simulink model "experimental_results"  (Simulink 10.2)
settings: Solver=ode1  StartTime=0.0  StopTime=60  FixedStep=0.002  RelTol=1e-3  EnableMultiTasking=on
PreLoadFcn:
  | quanser_aero_lqr
undefined symbols (not defined in the file or in its folder): HIL, qc_get_step_size
libraries: quarc_library x7
(part 1 of 2)
settings Model: Creator=MLevis  LastModifiedBy=ffsandva  SimulationMode=external  ExtModeTrigDuration=20000
settings SolverCC: PositivePriorityOrder=on
settings DataIOCC: LimitDataPoints=on  SignalLoggingSaveFormat=Dataset
settings DebuggingCC: UnderspecifiedInitializationDetection=Simplified  MergeDetectMultiDrivingBlocksExec=error  SolverPrmCheckMsg=warning  FcnCallInpInsideContextMsg=error
settings RTWCC: Description=QUARC Win64 Target  SystemTargetFile=quarc_win64.tlc  TemplateMakefile=quarc_default_tmf
settings STFCustomTargetCC: TargetPreCompLibLocation=C:\PROGRA~3\QUARC\lib\2020b\win64\release  ConcurrentExecutionCompliant=on  SystemTargetFile=quarc_win64.tlc
settings GRTTargetCC: TargetPreCompLibLocation=C:\PROGRA~3\QUARC\lib\2020b\win64\release  ParMdlRefBuildCompliant=off  CompOptLevelCompliant=off  MatFileLogging=off  CPPClassGenCompliant=off  UseToolchainInfoCompliant=off  ExtMode=on  ExtModeMexFile=quarc_comm
settings ConfigComp: CovSFcnEnable=off

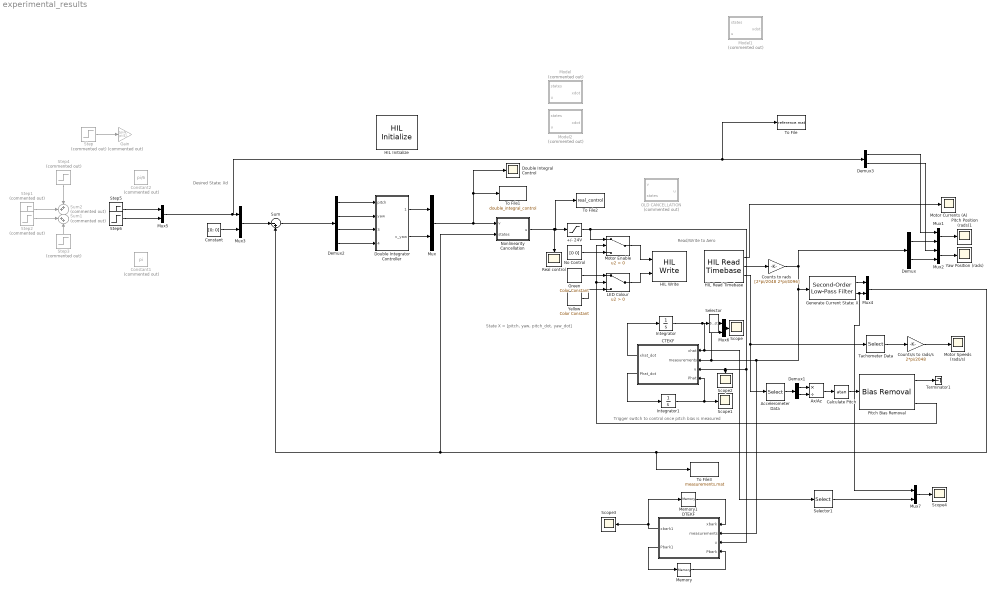
== system experimental_results ==
  note: Read/Write to Aero
  note: Trigger switch to control once pitch bias is measured
  note: Desired State; Xd
  note: State X = [pitch, yaw, pitch_dot, yaw_dot]
  +/- 24V : Saturate  UpperLimit=24  LowerLimit=-24
  Accelerometer Data : Selector  InputPortWidth=4  IndexOptions=Index vector (dialog)  Indices=[1 2]  OutputSizes=1
  Ax/Az : Product  Inputs=*/
  CTEKF : MATLAB Function  TreatAsAtomicUnit=on
  Calculate Pitch : Trigonometry  Operator=atan
  Constant : Constant  Value=[0; 0]
  Constant1 : Constant  Commented=on  Value=pi
  Constant2 : Constant  Commented=on  Value=pi/6
  Counts to rads : Gain  Gain=[2*pi/2048 2*pi/4096]
  Counts/s to rads/s : Gain  Gain=2*pi/2048
  DTEKF : MATLAB Function  TreatAsAtomicUnit=on
  Demux : Demux  Outputs=2
  Demux1 : Demux  Outputs=2
  Demux2 : Demux
  Demux3 : Demux  Outputs=2
  Double Integral Control : Scope
  Double Integrator Controller : Subsystem
  Gain : Gain  Commented=on  Gain=[pi/6; pi/4]
  Generate Current State; X : quarc_library/Continuous/Second-Order Low-Pass Filter  params_source=Internal (dialog parameters)  input_width=50  input_zeta=0.8  input_init=0
  Green : quarc_library/Sources/Signals/Color Constant  color=[0 1 0]
      settings: SourceProductName=QUARC Targets
  HIL Initialize : quarc_library/Data Acquisition/Generic/Configuration/HIL Initialize  Priority=-99  object_name=HIL-1  board_type=quanser_aero_usb  board_number=0  board_options=""  exclusive=off  active=off  hardware_clocks=[0]  clock_modes=[]  initial_clock_frequencies=[]  set_clock_params_at_start=off  set_clock_params_at_switch_in=off  set_clock_frequencies_at_start=off  set_clock_frequencies_at_switch_in=off  analog_input_channels=[0:1]  analog_input_configurations=[]  analog_input_maximums=3  analog_input_minimums=-3  set_analog_input_params_at_start=off  set_analog_input_params_at_switch_in=off  analog_output_channels=[0:1]  analog_output_maximums=24  analog_output_minimums=-24  initial_analog_outputs=[0]  final_analog_outputs=[0]  watchdog_analog_outputs=[0]  set_analog_output_params_at_start=off  set_analog_output_params_at_switch_in=off  set_analog_outputs_at_start=on  set_analog_outputs_at_switch_in=off  set_analog_outputs_at_terminate=on  set_analog_outputs_at_switch_out=off  set_analog_outputs_on_watchdog=on  digital_input_channels=[]  digital_output_channels=[0:1]  digital_output_configuration=[]  initial_digital_outputs=[1]  final_digital_outputs=[0]  watchdog_digital_outputs=[0]  set_digital_output_params_at_start=off  set_digital_output_params_at_switch_in=off  set_digital_outputs_at_start=on  set_digital_outputs_at_switch_in=off  set_digital_outputs_at_terminate=on  set_digital_outputs_at_switch_out=off  set_digital_outputs_on_watchdog=on  encoder_channels=[0:3]  quadrature=[4]  encoder_filter_frequency=[]  initial_encoder_counts=[0]  set_encoder_params_at_start=off  set_encoder_params_at_switch_in=off  set_encoder_counts_at_start=on  set_encoder_counts_at_switch_in=off  pwm_channels=[]  pwm_modes=[]  pwm_frequency=[]  pwm_configuration=[]  pwm_alignment=[]  pwm_polarity=[]  pwm_leading_deadband=[]  pwm_trailing_deadband=[]  initial_pwm_outputs=[]  final_pwm_outputs=[]  watchdog_pwm_outputs=[]  set_pwm_params_at_start=off  set_pwm_params_at_switch_in=off  set_pwm_outputs_at_start=off  set_pwm_outputs_at_switch_in=off  set_pwm_outputs_at_terminate=off  set_pwm_outputs_at_switch_out=off  set_pwm_outputs_on_watchdog=off  other_output_channels=[11000:11002]  initial_other_outputs=[0 1 0]  final_other_outputs=[1 0 0]  watchdog_other_outputs=[0 0 1]  set_other_outputs_at_start=on  set_other_outputs_at_switch_in=off  set_other_outputs_at_terminate=on  set_other_outputs_at_switch_out=off  set_other_outputs_on_watchdog=on
  HIL Read Timebase : quarc_library/Data Acquisition/Generic/Timebases/HIL Read Timebase  object_name=HIL-1  clock=0  analog_channels=[0:1]  encoder_channels=[2:3]  digital_channels=[]  other_channels=[4000 4002 14000 14001]  active=on  vector_output=on  data_type_mode=Inherit via back propagation  encoder_data_type=double  digital_data_type=boolean  overflow_mode=Error on overflow  samples_in_buffer=max(ceil(1/qc_get_step_size), 1)
  HIL Write : quarc_library/Data Acquisition/Generic/Immediate I//O/HIL Write  object_name=HIL-1  analog_channels=[0:1]  pwm_channels=[]  digital_channels=[]  other_channels=[11000:11002]  sample_time=-1  active=off  vector_input=on
  Integrator : Integrator  InitialCondition=[0;0;0;0]
  Integrator1 : Integrator  InitialCondition=zeros(4)
  LED Colour : Switch  Criteria=u2 > Threshold
  Memory : Memory  InitialCondition=zeros(4)
  Memory1 : Memory  InitialCondition=zeros(4,1)
  Model : MATLAB Function  Commented=on  TreatAsAtomicUnit=on
  Model1 : MATLAB Function  Commented=on  TreatAsAtomicUnit=on
  Model2 : MATLAB Function  Commented=on  TreatAsAtomicUnit=on
  Motor Currents (A) : Scope
  Motor Enable : Switch  Criteria=u2 > Threshold
  Motor Speeds (rads/s) : Scope
  Mux{,1..7} (8 alike) : Mux  Inputs=2
  No Control : Constant  Value=[0 0]
  Nonlinearity Cancellation : MATLAB Function  TreatAsAtomicUnit=on
  OLD CANCELLATION : MATLAB Function  Commented=on  TreatAsAtomicUnit=on
  Pitch Bias Removal : quarc_library/Discrete/Bias Removal  start_time=0  end_time=1  switch_id=0  sample_time=qc_get_step_size
      settings: SourceProductName=QUARC Targets
  Pitch Position (rads)1 : Scope
  Real control : Scope
  Scope{,1..4} (5 alike) : Scope
  Selector : Selector  InputPortWidth=4  IndexOptions=Index vector (dialog)  Indices=[1 2]  OutputSizes=1
  Selector1 : Selector  InputPortWidth=4  IndexOptions=Index vector (dialog)  Indices=[3 4]  OutputSizes=1
  Step : Step  Commented=on  Time=5  SampleTime=0
  Step1 : Step  Commented=on  Time=5  After=pi/6  SampleTime=0
  Step2 : Step  Commented=on  Time=5  After=-pi/2  SampleTime=0
  Step3 : Step  Commented=on  Time=30  After=pi/2  SampleTime=0
  Step4 : Step  Commented=on  Time=20  After=-pi/3  SampleTime=0
  Step5 : Step  Time=5  After=pi/6  SampleTime=0
  Step6 : Step  Time=5  After=pi/4  SampleTime=0
  Sum : Sum  Inputs=|-+
  Sum1 : Sum  Commented=on  Inputs=|++
  Sum2 : Sum  Commented=on  Inputs=++|
  Tachometer Data : Selector  InputPortWidth=4  IndexOptions=Index vector (dialog)  Indices=[3 4]  OutputSizes=1
  Terminator1 : Terminator
  To File : ToFile  Filename=reference.mat
  To File1 : ToFile  Filename=double_integral_control
  To File2 : ToFile  Filename=real_control
  To File3 : ToFile  Filename=measurements.mat
  Yaw Position (rads) : Scope
  Yellow : quarc_library/Sources/Signals/Color Constant  color=[1 1 0]
      settings: SourceProductName=QUARC Targets
  wires:
  HIL Read Timebase/2 -> Counts to rads/1
  +/- 24V/1 -> DTEKF/3(u), CTEKF/3(u), Scope2/1, Motor Enable/1
  Motor Enable/1 -> HIL Write/1
  Pitch Bias Removal/3 -> Motor Enable/2, LED Colour/2
  LED Colour/1 -> HIL Write/2
  No Control/1 -> Motor Enable/3
  Green/1 -> LED Colour/1
  Yellow/1 -> LED Colour/3
  Counts to rads/1 -> Demux/1, DTEKF/2(measurements), Mux6/2, CTEKF/2(measurements), Generate Current State; X/1
  HIL Read Timebase/3 -> Accelerometer Data/1, Tachometer Data/1
  Demux1/1 -> Ax/Az/1
  Demux1/2 -> Ax/Az/2
  Ax/Az/1 -> Calculate Pitch/1
  Calculate Pitch/1 -> Pitch Bias Removal/1
  Pitch Bias Removal/1 -> Terminator1/1
  HIL Read Timebase/1 -> Motor Currents (A)/1
  Counts/s to rads/s/1 -> Motor Speeds (rads/s)/1
  Tachometer Data/1 -> Counts/s to rads/s/1
  Accelerometer Data/1 -> Demux1/1
  Generate Current State; X/2 -> Mux7/1, Mux4/2
  Generate Current State; X/1 -> Mux4/1
  Demux/1 -> Mux1/2
  Mux1/1 -> Pitch Position (rads)1/1
  Demux/2 -> Mux2/2
  Mux2/1 -> Yaw Position (rads)/1
  Mux4/1 -> Sum/2, Nonlinearity Cancellation/2(states), To File3/1
  Double Integrator Controller/1(v_pitch) -> Mux/1
  Double Integrator Controller/2(v_yaw) -> Mux/2
  Demux2/1 -> Double Integrator Controller/1(pitch)
  Demux2/2 -> Double Integrator Controller/2(yaw)
  Demux2/3 -> Double Integrator Controller/3(pitch_dot)
  Demux2/4 -> Double Integrator Controller/4(yaw_dot)
  Sum/1 -> Demux2/1
  Mux5/1 -> To File/1, Demux3/1, Mux3/1
  Constant/1 -> Mux3/2
  Mux3/1 -> Sum/1
  Demux3/1 -> Mux1/1
  Demux3/2 -> Mux2/1
  Mux/1 -> Nonlinearity Cancellation/1(v), Double Integral Control/1, To File1/1
  Step/1 -> Gain/1
  Step2/1 -> Sum1/1
  Step1/1 -> Sum2/2
  Step3/1 -> Sum1/2
  Step4/1 -> Sum2/1
  Nonlinearity Cancellation/1(u) -> Real control/1, To File2/1, +/- 24V/1
  Step6/1 -> Mux5/2
  Step5/1 -> Mux5/1
  Integrator/1 -> Selector1/1, CTEKF/1(xhat), Selector/1
  CTEKF/2(Phat_dot) -> Integrator1/1
  Integrator1/1 -> Scope1/1, CTEKF/4(Phat)
  Mux6/1 -> Scope/1
  DTEKF/2(Pbark1) -> Memory/1
  Memory/1 -> DTEKF/4(Pbark)
  DTEKF/1(xbark1) -> Memory1/1, Scope3/1
  Memory1/1 -> DTEKF/1(xbark)
  Selector/1 -> Mux6/1
  Selector1/1 -> Mux7/2
  Mux7/1 -> Scope4/1
  CTEKF/1(xhat_dot) -> Integrator/1

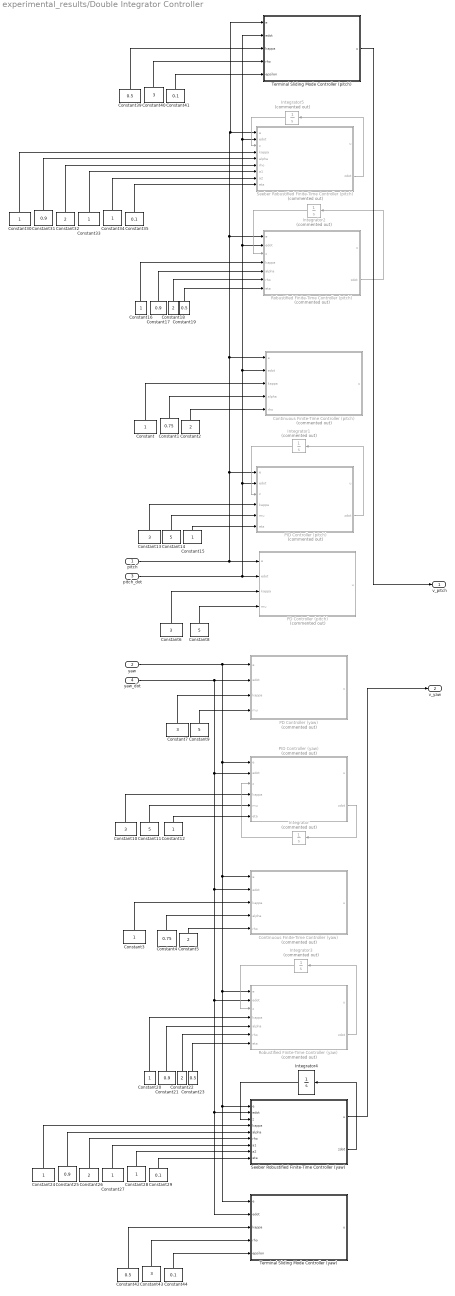
== system experimental_results/Double Integrator Controller ==
  pitch : Inport
  yaw : Inport  Port=2
  pitch_dot : Inport  Port=3
  yaw_dot : Inport  Port=4
  Constant{,3,12,15..16,20,24,27..28,30,33..34} (12 alike) : Constant
  Constant1 : Constant  Value=0.75
  Constant{6..7,10,13,40,43} (6 alike) : Constant  Value=3
  Constant{8..9,11,14} (4 alike) : Constant  Value=5
  Constant{17,21,25,31} (4 alike) : Constant  Value=0.9
  Constant{2,5,18,22,26,32} (6 alike) : Constant  Value=2
  Constant{19,23,39,42} (4 alike) : Constant  Value=0.5
  Constant{29,35,41,44} (4 alike) : Constant  Value=0.1
  Constant4 : Constant  Value=0.75
  Continuous Finite-Time Controller (pitch) : MATLAB Function  Commented=on  TreatAsAtomicUnit=on
  Continuous Finite-Time Controller (yaw) : MATLAB Function  Commented=on  TreatAsAtomicUnit=on
  Integrator{,1..3,5} (5 alike) : Integrator  Commented=on
  Integrator4 : Integrator
  PD Controller (pitch) : MATLAB Function  Commented=on  TreatAsAtomicUnit=on
  PD Controller (yaw) : MATLAB Function  Commented=on  TreatAsAtomicUnit=on
  PID Controller (pitch) : MATLAB Function  Commented=on  TreatAsAtomicUnit=on
  PID Controller (yaw) : MATLAB Function  Commented=on  TreatAsAtomicUnit=on
  Robustified Finite-Time Controller (pitch) : MATLAB Function  Commented=on  TreatAsAtomicUnit=on
  Robustified Finite-Time Controller (yaw) : MATLAB Function  Commented=on  TreatAsAtomicUnit=on
  Seeber Robustified Finite-Time Controller (pitch) : MATLAB Function  Commented=on  TreatAsAtomicUnit=on
  Seeber Robustified Finite-Time Controller (yaw) : MATLAB Function  TreatAsAtomicUnit=on
  Terminal Sliding Mode Controller (pitch) : MATLAB Function  TreatAsAtomicUnit=on
  Terminal Sliding Mode Controller (yaw) : MATLAB Function  TreatAsAtomicUnit=on
  v_pitch : Outport
  v_yaw : Outport  Port=2
  wires:
  pitch/1 -> Terminal Sliding Mode Controller (pitch)/1(e), Seeber Robustified Finite-Time Controller (pitch)/1(e), Robustified Finite-Time Controller (pitch)/1(e), Continuous Finite-Time Controller (pitch)/1(e), PID Controller (pitch)/1(e), PD Controller (pitch)/1(e)
  Constant/1 -> Continuous Finite-Time Controller (pitch)/3(kappa)
  Constant1/1 -> Continuous Finite-Time Controller (pitch)/4(alpha)
  Constant2/1 -> Continuous Finite-Time Controller (pitch)/5(rho)
  pitch_dot/1 -> PID Controller (pitch)/2(edot), Continuous Finite-Time Controller (pitch)/2(edot), Terminal Sliding Mode Controller (pitch)/2(edot), Seeber Robustified Finite-Time Controller (pitch)/2(edot), Robustified Finite-Time Controller (pitch)/2(edot), PD Controller (pitch)/2(edot)
  Constant3/1 -> Continuous Finite-Time Controller (yaw)/3(kappa)
  Constant5/1 -> Continuous Finite-Time Controller (yaw)/5(rho)
  Constant4/1 -> Continuous Finite-Time Controller (yaw)/4(alpha)
  yaw/1 -> Continuous Finite-Time Controller (yaw)/1(e), Terminal Sliding Mode Controller (yaw)/1(e), Seeber Robustified Finite-Time Controller (yaw)/1(e), Robustified Finite-Time Controller (yaw)/1(e), PID Controller (yaw)/1(e), PD Controller (yaw)/1(e)
  Constant6/1 -> PD Controller (pitch)/3(kappa)
  Constant8/1 -> PD Controller (pitch)/4(mu)
  Constant9/1 -> PD Controller (yaw)/4(mu)
  Constant7/1 -> PD Controller (yaw)/3(kappa)
  Constant10/1 -> PID Controller (yaw)/4(kappa)
  Constant11/1 -> PID Controller (yaw)/5(mu)
  PID Controller (yaw)/2(zdot) -> Integrator/1
  Integrator/1 -> PID Controller (yaw)/3(z)
  Constant12/1 -> PID Controller (yaw)/6(eta)
  yaw_dot/1 -> Continuous Finite-Time Controller (yaw)/2(edot), Robustified Finite-Time Controller (yaw)/2(edot), Terminal Sliding Mode Controller (yaw)/2(edot), Seeber Robustified Finite-Time Controller (yaw)/2(edot), PID Controller (yaw)/2(edot), PD Controller (yaw)/2(edot)
  PID Controller (pitch)/2(zdot) -> Integrator1/1
  Integrator1/1 -> PID Controller (pitch)/3(z)
  Constant13/1 -> PID Controller (pitch)/4(kappa)
  Constant14/1 -> PID Controller (pitch)/5(mu)
  Constant15/1 -> PID Controller (pitch)/6(eta)
  Robustified Finite-Time Controller (pitch)/2(zdot) -> Integrator2/1
  Integrator2/1 -> Robustified Finite-Time Controller (pitch)/3(z)
  Constant16/1 -> Robustified Finite-Time Controller (pitch)/4(kappa)
  Constant17/1 -> Robustified Finite-Time Controller (pitch)/5(alpha)
  Constant18/1 -> Robustified Finite-Time Controller (pitch)/6(rho)
  Constant19/1 -> Robustified Finite-Time Controller (pitch)/7(eta)
  Constant21/1 -> Robustified Finite-Time Controller (yaw)/5(alpha)
  Robustified Finite-Time Controller (yaw)/2(zdot) -> Integrator3/1
  Constant22/1 -> Robustified Finite-Time Controller (yaw)/6(rho)
  Constant23/1 -> Robustified Finite-Time Controller (yaw)/7(eta)
  Integrator3/1 -> Robustified Finite-Time Controller (yaw)/3(z)
  Constant20/1 -> Robustified Finite-Time Controller (yaw)/4(kappa)
  Seeber Robustified Finite-Time Controller (yaw)/2(zdot) -> Integrator4/1
  Constant27/1 -> Seeber Robustified Finite-Time Controller (yaw)/7(a1)
  Constant28/1 -> Seeber Robustified Finite-Time Controller (yaw)/8(a2)
  Constant25/1 -> Seeber Robustified Finite-Time Controller (yaw)/5(alpha)
  Constant24/1 -> Seeber Robustified Finite-Time Controller (yaw)/4(kappa)
  Constant26/1 -> Seeber Robustified Finite-Time Controller (yaw)/6(rho)
  Constant29/1 -> Seeber Robustified Finite-Time Controller (yaw)/9(eta)
  Integrator4/1 -> Seeber Robustified Finite-Time Controller (yaw)/3(z)
  Seeber Robustified Finite-Time Controller (pitch)/2(zdot) -> Integrator5/1
  Constant35/1 -> Seeber Robustified Finite-Time Controller (pitch)/9(eta)
  Constant32/1 -> Seeber Robustified Finite-Time Controller (pitch)/6(rho)
  Constant30/1 -> Seeber Robustified Finite-Time Controller (pitch)/4(kappa)
  Constant31/1 -> Seeber Robustified Finite-Time Controller (pitch)/5(alpha)
  Constant33/1 -> Seeber Robustified Finite-Time Controller (pitch)/7(a1)
  Integrator5/1 -> Seeber Robustified Finite-Time Controller (pitch)/3(z)
  Constant34/1 -> Seeber Robustified Finite-Time Controller (pitch)/8(a2)
  Constant41/1 -> Terminal Sliding Mode Controller (pitch)/5(epsilon)
  Constant40/1 -> Terminal Sliding Mode Controller (pitch)/4(rho)
  Constant39/1 -> Terminal Sliding Mode Controller (pitch)/3(kappa)
  Constant42/1 -> Terminal Sliding Mode Controller (yaw)/3(kappa)
  Constant44/1 -> Terminal Sliding Mode Controller (yaw)/5(epsilon)
  Constant43/1 -> Terminal Sliding Mode Controller (yaw)/4(rho)
  Seeber Robustified Finite-Time Controller (yaw)/1(u) -> v_yaw/1
  Terminal Sliding Mode Controller (pitch)/1(u) -> v_pitch/1

== matlab function Model2 ==
  data: xdot output double; states input double; u input double
function xdot = QuanserAeroModelModified(states, u)
    pitch = states(1);
%     yaw = states(2);
    pitch_dot = states(3);
    yaw_dot = states(4);

    g = 9.81;

    Jp = 2.15e-2;
    Jy = 2.37e-2;
    % dc = 3.25e-3;
    dc = 0.0071;
    dt = 0.158;
    mb = 1.075;
       
    Rm = 8.4;
    kt = 0.042;
    km = 0.042;
    kd = 1e-5;
    
    Kmp = 3.0633e-04;
    Kty = 6.1266e-04;
    Ktp = 5.8481e-04;
    Kmy = 7.5190e-04;
    
    k11 = 5.512e-05;
    k12 = 0.0001207;
    k21 = 4.131e-05;
    k22 = 0.0001915;
    
    M = [
        Jp + mb * dc^2, 0;
        0, Jy + mb * dc^2 * sin(pitch)^2;
    ];
    C = [
        0, -mb * dc^2 * yaw_dot * sin(pitch) * cos(pitch) - 0.5 * Jy * sin(pitch) * yaw_dot;
        2 * mb * dc^2 * yaw_dot * sin(pitch) * cos(pitch) - Jy * sin(pitch) * yaw_dot, 0;
    ];
    gvec = [
        mb * g * dc * sin(pitch);
        0;
    ];
%     B = dt * kt / (kt * km + kd * Rm) * [
%         Kmp, Ktp;
%         -Kmy, Kty;
%     ];
    B = [
        0.0011, 0.0021;
        -0.0027, 0.0022;
    ];
    qdot = [
        pitch_dot;
        yaw_dot;
    ];
    D = [
        0.00711, 0;
        0, 0.0220;
    ];
    b = [
        k11 * u(1) + k12 * u(1)^2 + k21 * u(2) + k22 * u(2)^2;
        -k21 * u(1) - k22 * u(1)^2 + k11 * u(2) + k12 * u(2)^2;
    ];

    xdot = [
        qdot;
        M \ (b - C * qdot - gvec - D * qdot);
    ];
end

== matlab function Model ==
  data: states input double; u input double; xdot output double
function xdot = QuanserAeroModel(states, u)
    pitch = states(1);
%     yaw = states(2);
    pitch_dot = states(3);
    yaw_dot = states(4);

    g = 9.81;

    Jp = 2.15e-2;
    Jy = 2.37e-2;
    % dc = 3.25e-3;
    dc = 0.0071;
    dt = 0.158;
    mb = 1.075;
       
    Rm = 8.4;
    kt = 0.042;
    km = 0.042;
    kd = 1e-5;
    
    Kmp = 3.0633e-04;
    Kty = 6.1266e-04;
    Ktp = 5.8481e-04;
    Kmy = 7.5190e-04;
    
    k11 = 5.512e-05;
    k12 = 0.0001207;
    k21 = 4.131e-05;
    k22 = 0.0001915;
    
    M = [
        Jp + mb * dc^2, 0;
        0, Jy + mb * dc^2 * sin(pitch)^2;
    ];
    C = [
        0, -mb * dc^2 * yaw_dot * sin(pitch) * cos(pitch);
        2 * mb * dc^2 * yaw_dot * sin(pitch) * cos(pitch), 0;
    ];
    gvec = [
        mb * g * dc * sin(pitch);
        0;
    ];
%     B = dt * kt / (kt * km + kd * Rm) * [
%         Kmp, Ktp;
%         -Kmy, Kty;
%     ];
    B = [
        0.0011, 0.0021;
        -0.0027, 0.0022;
    ];
    qdot = [
        pitch_dot;
        yaw_dot;
    ];
    D = [
        0.00711, 0;
        0, 0.0220;
    ];
    b = [
        k11 * u(1) + k12 * u(1)^2 + k21 * u(2) + k22 * u(2)^2;
        -k21 * u(1) - k22 * u(1)^2 + k11 * u(2) + k12 * u(2)^2;
    ];

    xdot = [
        qdot;
        % M \ (B * u - C * qdot - gvec - D * qdot);
        M \ (b - C * qdot - gvec - D * qdot);
    ];
end

== matlab function Model1 ==
  data: states input double; u input double; xdot output double
function xdot = QuanserAeroKumar(states, u)
    pitch = states(1);
%     yaw = states(2);
    pitch_dot = states(3);
    yaw_dot = states(4);

    g = 9.81;

    Jp = 2.15e-2;
    Jy = 2.37e-2;
    dc = 3.25e-3;
    dt = 0.158;
    mb = 1.075;
       
    Rm = 8.4;
    kt = 0.042;
    km = 0.042;
    kd = 1e-5;
    
    Kpp = 0.0011;                                                                                                                                                                                                                                                                                                                                                                                                                                                                                                                                                                                                                                                                                                                                                                                                                                                                                                                                                                                                                                                                                                                                                                                                                                                                                                                                                                                                                                                                                                                                                                                                                                                                                                                                                                                                                                                                                                                                                                                                                                                                                                                                                                                                                                                                                                                                                                                                                                                                                                                                                                                                                                                                                                                                                                                                                                                                                                                                                                                                                                                                                                                                                                                                                                                                                                                                                                                                                                                                                                                                                                                                                                                                                                                                                                                                                                                                                                                                                                                                                                                                                                                                                                                                                                                                                                                                                                                                                                                                                                                                                                                                                                                                                                                                                                                                                                                                                                                                                                                                                                                                                                                                                                                                                                                                                                                                                                                                                                                                                                                                                                                                                                                                                                                                                                                                                                                                                                                                                                                                                                                                                                                                                                                                                                                                                                                                                                                                                                                                                                                                                                                                                                                                                                                                                                                                                                                                                                                                                                                                                                                                                                                                                                                                                                                                                                                                                                                                                                                                                                                                                                                                                                                                                                                                                                                                                                                                                                                                                                                                                                                                                                                                                                                                                                                                                                                                                                                                                                                                                                                                                                                                                                                                                                                                                                                                                                                                                                                                                                                                                                                                                                                                                                                                                                                                                                                                                                                                                                                                                                                                                                                                                                                                                                                                                                                                                                                                                                                                                                                                                                                                                                                                                                                                                                                                                                                                                                                                                                                                                                                                                                              
    Kpy = 0.0021;
    Kyp = -0.0027;
    Kyy = 0.0022;
    
    Jeqp = 0.0219;
    Jeqy = 0.0220;
    Bp = 0.00711;
    By = 0.0220;
    l = 0.0071;
    m = 1.0750;
    
    a = Jeqp + m * l^2;
    b = Jeqy + m * l^2 * cos(pitch)^2;

    xdot = [
       pitch_dot;
       yaw_dot;
       (Kpp * u(1) + Kpy * u(2) - Bp * pitch_dot - m*g*l*cos(pitch) - m*l^2*sin(pitch)*cos(pitch)*yaw_dot^2)/a;
       (Kyp * u(1) + Kyy * u(2) - By * yaw_dot + 2*m*l^2*sin(pitch)*cos(pitch)*pitch_dot*yaw_dot)/b;
    ];
end

== matlab function Nonlinearity Cancellation ==
  data: v input double; states input double; u output double
function u = NonlinearityCancellation(v, states)
    theta = states(1);
    psi = states(2);
    thetadot = states(3);
    psidot = states(4);
    
    % parameters
    g = 9.81;
    dt = 0.158;
    me = 0.2;
    dx = 0.016;
    
    ry = 0.02;
    my = 0.526;
    
    mpa = 0.146;
    lt = 0.165;
    mmt = 0.089;
    mtt = 0.089;
    mtc = 0.280;
    mrod = mmt + mtt + mtc;
    
    Ibyy = 2*mpa*dt^2 + 2*me*dt^2 + me*dx^2 + 1/12*mrod*lt^2;
    Ifyzz = 1/2*my*ry^2;
    
    M = [
        Ibyy, 0;
        0, Ifyzz + Ibyy * cos(theta)^2;
    ];
    C = [
        0, Ibyy * psidot * cos(theta)*sin(theta);
        0, -2*Ibyy * thetadot * cos(theta)*sin(theta);
    ];
    gvec = [
        dx * g * me * sin(theta);
        0;
    ];
    
    Kmtheta = 1.26e-6;
    Kttheta = 1.08e-6;
    Kmpsi = Kttheta;
    Ktpsi = Kmtheta; 

    K_omega = 17.38;
    
    B = K_omega^2 * dt * [
        Kmtheta, Kttheta;
        -Kmpsi * cos(theta), Ktpsi * cos(theta);
    ];

    d1 = 0.0031;
    d2 = 0.0075;

    D = [
        d1, 0;
        0, d2;
    ];

    q = [
        theta;
        psi;
    ];
    qdot = [
        thetadot;
        psidot;
    ];

    utilde = B \ (M*v + C * qdot + D * qdot + gvec);
    u = sign(utilde) .* sqrt(abs(utilde));
end

== matlab function Double Integrator Controller/Continuous Finite-Time Controller (yaw) ==
  data: e input double; u output double; edot input double; kappa input double; alpha input double; rho input double
function u = ContinuousFiniteTimeController(e, edot, kappa, alpha, rho)
    % u = OrbitalTerminalSlidingMode(e, edot, kappa, alpha, rho) computes
    % the feedback control for a continuous finite-time controller given 
    % the positive parameters kappa, alpha and rho.
    %
    % Author:   Finn F. Sandvand
    % Date:     15th Jun 2025
    % Revisions: 

    sigma = edot + kappa * sign(e) * abs(e)^alpha;
    mu = alpha * kappa^(1/alpha) + rho;
    u = alpha * kappa^2 * sign(e) * abs(e)^(2*alpha-1) ...
        - mu * sign(sigma) * abs(sigma)^((2*alpha-1)/alpha);
end

== matlab function Double Integrator Controller/PD Controller (pitch) ==
  data: e input double; u output double; edot input double; kappa input double; mu input double
function u = PDController(e, edot, kappa, mu)
    % u = PDController(e, edot, kappa, mu) computes the feedback control 
    % for a Proportional-Derivative controller given the positive 
    % parameters kappa and mu.
    %
    % Author:   Finn F. Sandvand
    % Date:     15th Jun 2025
    % Revisions: 

    if kappa <= 0 || mu <= 0
        error('Error. kappa and mu must be positive');
    elseif kappa >= mu
        error('Error. kappa must be greater than mu');
    end

    sigma = edot + kappa * e;
    u = kappa^2 * e - mu * sigma;
end

== matlab function Double Integrator Controller/PD Controller (yaw) ==
  data: e input double; u output double; edot input double; kappa input double; mu input double
function u = PDController(e, edot, kappa, mu)
    % u = PDController(e, edot, kappa, mu) computes the feedback control 
    % for a Proportional-Derivative controller given the positive 
    % parameters kappa and mu.
    %
    % Author:   Finn F. Sandvand
    % Date:     15th Jun 2025
    % Revisions: 

    if kappa <= 0 || mu <= 0
        error('Error. kappa and mu must be positive');
    elseif kappa >= mu
        error('Error. kappa must be greater than mu');
    end

    sigma = edot + kappa * e;
    u = kappa^2 * e - mu * sigma;
end

== matlab function Double Integrator Controller/PID Controller (yaw) ==
  data: e input double; u output double; edot input double; z input double; kappa input double; mu input double; eta input double; zdot output double
function [u, zdot] = PIDController(e, edot, z, kappa, mu, eta)
    % [u, zdot] = RobustifiedFiniteTimeController(e, edot, z, kappa, mu, eta) 
    % computes the feedback control for a Proportional-Integral-Derviative
    % controller given the positive parameters kappa, mu and eta.
    %
    % Author:   Finn F. Sandvand
    % Date:     15th Jun 2025
    % Revisions: 

    if kappa <= 0 || mu <= 0 || eta <= 0
        error('Error. kappa, mu and eta must be positive');
    elseif kappa >= mu
        error('Error. kappa must be greater than mu');
    end

    sigma = edot + kappa * e;
    u = -kappa*(mu - kappa) * e - mu * edot - eta * z;
    zdot = sigma;
end

== matlab function Double Integrator Controller/PID Controller (pitch) ==
  data: e input double; u output double; edot input double; z input double; kappa input double; mu input double; eta input double; zdot output double
function [u, zdot] = PIDController(e, edot, z, kappa, mu, eta)
    % [u, zdot] = RobustifiedFiniteTimeController(e, edot, z, kappa, mu, eta) 
    % computes the feedback control for a Proportional-Integral-Derviative
    % controller given the positive parameters kappa, mu and eta.
    %
    % Author:   Finn F. Sandvand
    % Date:     15th Jun 2025
    % Revisions: 

    if kappa <= 0 || mu <= 0 || eta <= 0
        error('Error. kappa, mu and eta must be positive');
    elseif kappa >= mu
        error('Error. kappa must be greater than mu');
    end

    sigma = edot + kappa * e;
    u = -kappa*(mu - kappa) * e - mu * edot - eta * z;
    zdot = sigma;
end

== matlab function Double Integrator Controller/Continuous Finite-Time Controller (pitch) ==
  data: e input double; u output double; edot input double; kappa input double; alpha input double; rho input double
function u = ContinuousFiniteTimeController(e, edot, kappa, alpha, rho)
    % u = OrbitalTerminalSlidingMode(e, edot, kappa, alpha, rho) computes
    % the feedback control for a continuous finite-time controller given 
    % the positive parameters kappa, alpha and rho.
    %
    % Author:   Finn F. Sandvand
    % Date:     15th Jun 2025
    % Revisions: 

    sigma = edot + kappa * sign(e) * abs(e)^alpha;
    mu = alpha * kappa^(1/alpha) + rho;
    u = alpha * kappa^2 * sign(e) * abs(e)^(2*alpha-1) ...
        - mu * sign(sigma) * abs(sigma)^((2*alpha-1)/alpha);
end

== matlab function Double Integrator Controller/Robustified Finite-Time Controller (pitch) ==
  data: e input double; u output double; edot input double; z input double; kappa input double; alpha input double; rho input double; zdot output double; eta input double
function [u, zdot] = RobustifiedFiniteTimeController(e, edot, z, kappa, alpha, rho, eta)
    % [u, zdot] = RobustifiedFiniteTimeController(e, edot, z, kappa, alpha, rho, eta) 
    % computes the feedback control for a robustified finite-time
    % controller given the positive parameters kappa, alpha, rho and eta.
    %
    % Author:   Finn F. Sandvand
    % Date:     15th Jun 2025
    % Revisions: 

    sigma = edot + kappa * sign(e) * abs(e)^alpha;
    mu = alpha * kappa^(1/alpha) + rho;
    u = alpha * kappa^2 * sign(e) * abs(e)^(2*alpha-1) ...
        - mu * sign(sigma) * abs(sigma)^((2*alpha-1)/alpha) - eta * z;
    zdot = sign(sigma);
end

== matlab function Double Integrator Controller/Robustified Finite-Time Controller (yaw) ==
  data: e input double; u output double; edot input double; z input double; kappa input double; alpha input double; rho input double; zdot output double; eta input double
function [u, zdot] = RobustifiedFiniteTimeController(e, edot, z, kappa, alpha, rho, eta)
    % [u, zdot] = RobustifiedFiniteTimeController(e, edot, z, kappa, alpha, rho, eta) 
    % computes the feedback control for a robustified finite-time
    % controller given the positive parameters kappa, alpha, rho and eta.
    %
    % Author:   Finn F. Sandvand
    % Date:     15th Jun 2025
    % Revisions: 

    sigma = edot + kappa * sign(e) * abs(e)^alpha;
    mu = alpha * kappa^(1/alpha) + rho;
    u = alpha * kappa^2 * sign(e) * abs(e)^(2*alpha-1) ...
        - mu * sign(sigma) * abs(sigma)^((2*alpha-1)/alpha) - eta * z;
    zdot = sign(sigma);
end

== matlab function Double Integrator Controller/Seeber Robustified Finite-Time Controller (yaw) ==
  data: e input double; u output double; edot input double; z input double; kappa input double; alpha input double; rho input double; zdot output double; a1 input double; a2 input double; eta input double
function [u, zdot] = SeeberRobustifiedFiniteTimeController(e, edot, z, kappa, alpha, rho, a1, a2, eta)
    % [u, zdot] = SeeberRobustifiedFiniteTimeController(e, edot, z, kappa, alpha, rho, a1, a2, eta) 
    % computes the feedback control for a robustified finite-time
    % controller given the positive parameters kappa, alpha, rho, a1, a2
    % and eta.
    %
    % Author:   Finn F. Sandvand
    % Date:     15th Jun 2025
    % Revisions: 

    sigma = edot + kappa * sign(e) * abs(e)^alpha;
    mu = alpha * kappa^(1/alpha) + rho;
    k = alpha * kappa^2 * sign(e) * abs(e)^(2*alpha-1) ...
        - mu * sign(sigma) * abs(sigma)^((2*alpha-1)/alpha);

    h = edot / (a1 * abs(e)^(2-alpha) + a2 * abs(edot)^((2-alpha)/alpha))^((2*alpha-1)/(2-alpha));
    dhdx1 = a1 * (1-2*alpha) * abs(e)^(1-alpha) * edot / (a1 * abs(e)^(2-alpha) + a2 * abs(edot)^((2-alpha)/alpha))^((alpha+1)/(2-alpha));
    dhdx2 = 1 / (a1 * abs(e)^(2-alpha) + a2 * abs(edot)^((2-alpha)/alpha))^((2*alpha-1)/(2-alpha)) + a2 * (1-2*alpha)/alpha * sign(edot) * abs(edot)^(1/alpha) / (a1 * abs(e)^(2-alpha) + a2 * abs(edot)^((2-alpha)/alpha))^((alpha+1)/(2-alpha));

    % handle singular cases
    if isnan(dhdx1)
        dhdx1 = 0;
    end
    if isnan(dhdx2)
        dhdx2 = 0;
    end
    if isnan(h)
        h = 0;
    end

    u = k - eta * h + eta * z;
    zdot = dhdx1 * edot + dhdx2 * k;
end

== matlab function Double Integrator Controller/Seeber Robustified Finite-Time Controller (pitch) ==
  data: e input double; u output double; edot input double; z input double; kappa input double; alpha input double; rho input double; zdot output double; a1 input double; a2 input double; eta input double
function [u, zdot] = SeeberRobustifiedFiniteTimeController(e, edot, z, kappa, alpha, rho, a1, a2, eta)
    % [u, zdot] = SeeberRobustifiedFiniteTimeController(e, edot, z, kappa, alpha, rho, a1, a2, eta) 
    % computes the feedback control for a robustified finite-time
    % controller given the positive parameters kappa, alpha, rho, a1, a2
    % and eta.
    %
    % Author:   Finn F. Sandvand
    % Date:     15th Jun 2025
    % Revisions: 

    sigma = edot + kappa * sign(e) * abs(e)^alpha;
    mu = alpha * kappa^(1/alpha) + rho;
    k = alpha * kappa^2 * sign(e) * abs(e)^(2*alpha-1) ...
        - mu * sign(sigma) * abs(sigma)^((2*alpha-1)/alpha);

    h = edot / (a1 * abs(e)^(2-alpha) + a2 * abs(edot)^((2-alpha)/alpha))^((2*alpha-1)/(2-alpha));
    dhdx1 = a1 * (1-2*alpha) * abs(e)^(1-alpha) * edot / (a1 * abs(e)^(2-alpha) + a2 * abs(edot)^((2-alpha)/alpha))^((alpha+1)/(2-alpha));
    dhdx2 = 1 / (a1 * abs(e)^(2-alpha) + a2 * abs(edot)^((2-alpha)/alpha))^((2*alpha-1)/(2-alpha)) + a2 * (1-2*alpha)/alpha * sign(edot) * abs(edot)^(1/alpha) / (a1 * abs(e)^(2-alpha) + a2 * abs(edot)^((2-alpha)/alpha))^((alpha+1)/(2-alpha));

    % handle singular cases
    if isnan(dhdx1)
        dhdx1 = 0;
    end
    if isnan(dhdx2)
        dhdx2 = 0;
    end
    if isnan(h)
        h = 0;
    end

    u = k - eta * h + eta * z;
    zdot = dhdx1 * edot + dhdx2 * k;
end

== matlab function CTEKF ==
  data: xhat input double; measurements input double; xhat_dot output double; u input double; Phat input double; Phat_dot output double
function [xhat_dot, Phat_dot] = ExtendedKalmanFilter(xhat, measurements, u, Phat)
    theta = xhat(1);
    psi = xhat(2);
    thetadot = xhat(3);
    psidot = xhat(4);
    
    utilde = u.^2;
    utilde1 = utilde(1);
    utilde2 = utilde(2);
    
    R = diag([2.36e-6; 5.8974e-07]);
    Q = diag([0; 0; 1; 1]);

    % parameters
    g = 9.81;
    dt = 0.158;
    me = 0.2;
    dx = 0.016;
    
    ry = 0.02;
    my = 0.526;
    
    mpa = 0.146;
    lt = 0.165;
    mmt = 0.089;
    mtt = 0.089;
    mtc = 0.280;
    mrod = mmt + mtt + mtc;
    
    Ibyy = 2*mpa*dt^2 + 2*me*dt^2 + me*dx^2 + 1/12*mrod*lt^2;
    Ifyzz = 1/2*my*ry^2;

%     kt = 0.042;
%     km = 0.042;
%     kd = 1e-5;
%     Rm = 8.4;
    
    % Komega = kt / (kt * km + kd * Rm);
    Komega = 17.38;
    
%     Kmtheta = 1.58e-6;
%     Kttheta = 1.35e-6;
    Kmtheta = 1.26e-6;
    Kttheta = 1.08e-6;
    Kmpsi = Kttheta;
    Ktpsi = Kmtheta; 
%     Kmpsi = 4.81e-07;
%     Ktpsi = 6.88e-07; 
    
%     d1 = 0.00711;
%     d2 = 0.0220;
    d1 = 0.0031;
    d2 = 0.0075;

    F = [
                                                                                                                                                                                                                                                                                                                                                                                           0, 0,                                                                 1,                                                              0;
                                                                                                                                                                                                                                                                                                                                                                                           0, 0,                                                                 0,                                                              1;
                                                                                                                                                                                                                                                                                                                             -(Ibyy*(2*cos(theta)^2 - 1)*psidot^2 + dx*g*me*cos(theta))/Ibyy, 0,                                                          -d1/Ibyy,                                           -psidot*sin(2*theta);
        (4*Ibyy*psidot*thetadot*(2*cos(theta)^2 - 1) + 2*Kmpsi*Komega^2*dt*utilde1*sin(theta) - 2*Komega^2*Ktpsi*dt*utilde2*sin(theta))/(Ibyy + 2*Ifyzz + Ibyy*(2*cos(theta)^2 - 1)) - (2*Ibyy*cos(theta)*sin(theta)*(d2*psidot + Kmpsi*Komega^2*dt*utilde1*cos(theta) - Komega^2*Ktpsi*dt*utilde2*cos(theta) - 2*Ibyy*psidot*thetadot*cos(theta)*sin(theta)))/(Ibyy*cos(theta)^2 + Ifyzz)^2, 0, (2*Ibyy*psidot*cos(theta)*sin(theta))/(Ibyy*cos(theta)^2 + Ifyzz), -(d2 - Ibyy*thetadot*sin(2*theta))/(Ibyy*cos(theta)^2 + Ifyzz);
    ];
    H = [eye(2), zeros(2)];
    h = H * xhat;

    M = [
        Ibyy, 0;
        0, Ifyzz + Ibyy * cos(theta)^2;
    ];
    C = [
        0, Ibyy * psidot * cos(theta)*sin(theta);
        0, -2*Ibyy * thetadot * cos(theta)*sin(theta);
    ];
    gvec = [
        dx * g * me * sin(theta);
        0;
    ];
    B = Komega^2 * dt * [
        Kmtheta, Kttheta;
        -Kmpsi * cos(theta), Ktpsi * cos(theta);
    ];
    D = [
        d1, 0;
        0, d2;
    ];
    qdot = [
        thetadot;
        psidot;
    ];
    
    f = [
        qdot;
        M \ (B*utilde - C*qdot - gvec - D*qdot);
    ];
    

    K = Phat * H' / R;
    xhat_dot = f + K * (measurements - h);
    Phat_dot = F * Phat + Phat * F' + Q - K * H * Phat;
end
